simulink library "FloatLibraryOldBlocksBackup"  (R2019a)
settings: Solver=VariableStepAuto  StartTime=0.0  StopTime=10.0  RelTol=1e-3
libraries: arduinolib x2, dspstat3 x2, $bdroot x1
settings Model: Creator=Peter  LastModifiedBy=Peter

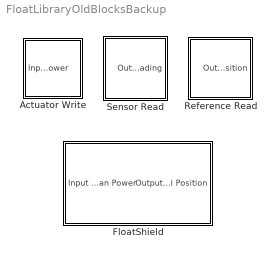
== system FloatLibraryOldBlocksBackup ==
  Actuator Write : Subsystem
      mask DialogControl DescGroupVar Prompt: FloatShield Fan
      mask DialogControl DescTextVar Prompt: Sets power level to the rotating fan at the bottom of the FloatShield tube. Expects input in form of percentual value from 0% to 100%.
      mask Display: image('assets\Fan.svg');
  FloatShield : Subsystem  mask{OutRadio=Percentage (%), Tcal=10, Ts=0.025}
      mask prompts: OutRadio "Output type"; Tcal "Calibration time (s):"; Ts "Sampling period (s):"
      mask init:
      | if OutRadio==1
      |     SatMin=0;
      |     SatMax=100;
      | else
      |     SatMin=0;
      |     SatMax=350;
      | end
      mask TypeOptions OutRadio: Percentage (%) | Altitude (mm)
      mask DialogControl DescGroupVar Prompt: FloatShield
      mask DialogControl DescTextVar Prompt: The block represents the FloatShield device. It accepts an input signal in the range of 0-100% that controls the fan power level and outputs ball position in form selected by the user. The block requires a sampling period and a calibration time at the beginning of the experiment to find out the reading extreme values.
      mask Display: image('assets\FloatShield.svg');
  Reference Read : Subsystem  mask{ReadoutRadio=Percentage (%), Ts=0.025}
      mask prompts: ReadoutRadio "Readout type"; Ts "Sampling period (s):"
      mask init:
      | if ReadoutRadio==1 
      | GainVal = (100/1023);                               
      | elseif ReadoutRadio==2
      | GainVal = (5/1023);                     
      | else
      | GainVal = 1;             
      | end
      mask TypeOptions ReadoutRadio: Percentage (%) | Voltage (V) | Analog value (ADC)
      mask DialogControl DescGroupVar Prompt: FloatShield Potentiometer
      mask DialogControl DescTextVar Prompt: The block represents potentiometer runner on the FloatShield device. User can choose the form of block output that represents the current potentiometer runner position.
      mask Display: image('assets\Potentiometer.svg');
  Sensor Read : Subsystem  mask{OutRadio=Distance (mm), CalType=Default values (recommended), MinVal=15, MaxVal=345, Ts=0.025}
      mask prompts: OutRadio "Output type"; CalType "Calibration values:"; MinVal "Minimal reading (mm):"; MaxVal "Maximal reading (mm):"; Ts "Sampling period (s):"
      mask init:
      | if CalType==1
      |     MinVal=15;
      |     MaxVal=345;
      | end
      | 
      | if OutRadio==2
      |     Rng=MaxVal-MinVal;    
      |     SatMin=0;
      |     SatMax=MaxVal;    
      | else   
      |     Rng=100;
      |     SatMin=0;
      |     SatMax=100;
      | end
      mask TypeOptions OutRadio: Distance (mm) | Altitude (mm) | Percentage (%)
      mask Callback OutRadio:
      | CurrentBlock = gcb;
      | Output = get_param(CurrentBlock,'OutRadio')
      | Calib = get_param(CurrentBlock,'CalType')
      | Menu = Simulink.Mask.get(CurrentBlock);
      | CalibOpt = Menu.getParameter('CalType')
      | MinOpt = Menu.getParameter('MinVal');
      | MaxOpt = Menu.getParameter('MaxVal')
      | 
      | if strcmp(Output,'Distance (mm)')
      | CalibOpt.Enabled='off';
      | MinOpt.Enabled='off';
      | MaxOpt.Enabled='off';
      | elseif strcmp(Calib,'Manual values')
      | CalibOpt.Enabled='on';
      | MinOpt.Enabled='on';
      | MaxOpt.Enabled='on';
      | else
      | CalibOpt.Enabled='on';
      | MinOpt.Enabled='off';
      | MaxOpt.Enabled='off';
      | end
      mask TypeOptions CalType: Default values (recommended) | Manual values
      mask Callback CalType:
      | CurrentBlock = gcbh;
      | Output = get_param(CurrentBlock,'OutRadio');
      | Calib = get_param(CurrentBlock,'CalType');
      | Menu = Simulink.Mask.get(CurrentBlock);
      | MinOpt = Menu.getParameter('MinVal');
      | MaxOpt = Menu.getParameter('MaxVal');
      | 
      | if strcmp(Output,'Distance (mm)')
      | MinOpt.Enabled='off';
      | MaxOpt.Enabled='off';
      | elseif strcmp(Calib,'Manual values')
      | MinOpt.Enabled='on';
      | MaxOpt.Enabled='on';
      | else
      | MinOpt.Enabled='off';
      | MaxOpt.Enabled='off';
      | end
      mask DialogControl DescGroupVar Prompt: FloatShield Distance Sensor
      mask DialogControl DescTextVar Prompt: The block represents the I2C Time of Flight VL53L0X Distance Sensor on the FloatShield device. User can choose type of reading this block outputs. For Altitude or Percentage output, calibration values are required. By default the most probable values are used, but if needed they can be manually set. User can also specify sampling period in seconds.
      mask DialogControl MinVal Tooltip: Recommended 15 mm.
      mask DialogControl MaxVal Tooltip: Recommended 345 mm.
      mask Display: image('assets\TOF.svg');

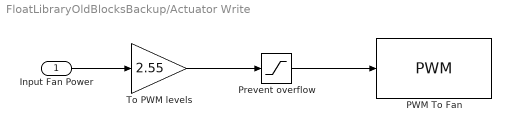
== system FloatLibraryOldBlocksBackup/Actuator Write ==
  Input Fan Power : Inport
  PWM To Fan : arduinolib/PWM  pinNumber=3  EnableInputFrequency=off  InitialFrequency=2000  InitialDutyCycle=0  NotificationType=None  blockPlatform=arduino
  Prevent overflow : Saturate  UpperLimit=255  LowerLimit=0
  To PWM levels : Gain  Gain=2.55
  wires:
  Prevent overflow/1 -> PWM To Fan/1
  To PWM levels/1 -> Prevent overflow/1
  Input Fan Power/1 -> To PWM levels/1

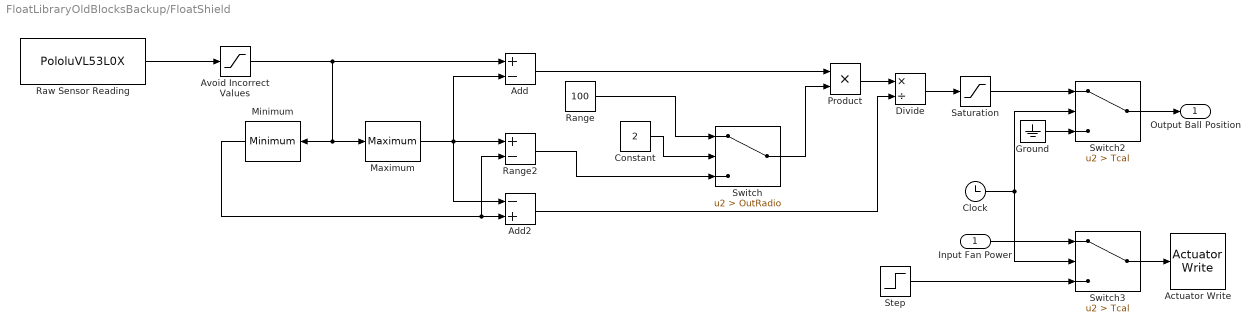
== system FloatLibraryOldBlocksBackup/FloatShield ==
  Input Fan Power : Inport
  Actuator Write : $bdroot/Actuator Write
  Add : Sum  Inputs=+-
  Add2 : Sum  Inputs=-+
  Avoid Incorrect Values : Saturate  UpperLimit=345  LowerLimit=15
  Clock : Clock
  Constant : Constant  Value=2  SampleTime=Ts
  Divide : Product  Inputs=*/
  Ground : Ground
  Maximum : dspstat3/Maximum  operation=maximum  fcn=Running  indexBase=One  operateOver=Each column  Dimension=1  reset=None  roiEnable=off  roiType=Rectangles  roiPortion=Entire ROI  roiOutput=Individual statistics for each ROI  roiFlag=off  roundingMode=Floor  overflowMode=off  accumDataTypeStr=Inherit: Same as product output  accumLastDataTypeStr=Inherit: Same as product output
  Minimum : dspstat3/Minimum  operation=minimum  fcn=Running  indexBase=One  operateOver=Each column  Dimension=1  reset=None  roiEnable=off  roiType=Rectangles  roiPortion=Entire ROI  roiOutput=Individual statistics for each ROI  roiFlag=off  roundingMode=Floor  overflowMode=off
      settings: SourceProductName=DSP System Toolbox  SourceProductBaseCode=DS
  Product : Product
  Range : Constant  Value=100  SampleTime=Ts
  Range2 : Sum  Inputs=+-
  Raw Sensor Reading : S-Function  FunctionName=PololuVL53L0X  SFunctionModules='PololuVL53L0X_wrapper'  SFunctionDeploymentMode=off  EnableBusSupport=off
  Saturation : Saturate  UpperLimit=SatMax  LowerLimit=SatMin
  Step : Step  Time=round((Tcal/2)/Ts)*Ts  After=100  SampleTime=Ts
  Switch : Switch  Criteria=u2 > Threshold  Threshold=OutRadio
  Switch2 : Switch  Criteria=u2 > Threshold  Threshold=Tcal
  Switch3 : Switch  Criteria=u2 > Threshold  Threshold=Tcal
  Output Ball Position : Outport
  wires:
  Range/1 -> Switch/1
  Range2/1 -> Switch/3
  Constant/1 -> Switch/2
  Switch2/1 -> Output Ball Position/1
  Input Fan Power/1 -> Switch3/1
  Switch3/1 -> Actuator Write/1
  Ground/1 -> Switch2/3
  Product/1 -> Divide/1
  Saturation/1 -> Switch2/1
  Avoid Incorrect Values/1 -> Add/1, Maximum/1, Minimum/1
  Add2/1 -> Divide/2
  Divide/1 -> Saturation/1
  Raw Sensor Reading/1 -> Avoid Incorrect Values/1
  Step/1 -> Switch3/3
  Minimum/1 -> Add2/2, Range2/2
  Clock/1 -> Switch3/2, Switch2/2
  Maximum/1 -> Add2/1, Add/2, Range2/1
  Add/1 -> Product/1
  Switch/1 -> Product/2

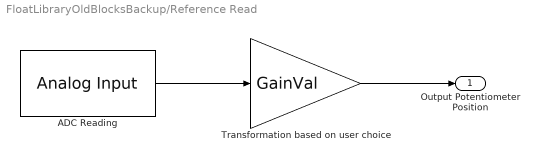
== system FloatLibraryOldBlocksBackup/Reference Read ==
  ADC Reading : arduinolib/Analog Input  pinNumber=0  ReadResultsOnly=off  ConversionTriggerSource=Software  ExternalTriggerType=uint32(0)  OutputDataType=uint16  EnableConversionCompleteNotify=off  EnableOuputStatus=off  SampleTime=Ts  blockPlatform=arduino
  Transformation based on user choice : Gain  Gain=GainVal  ParamDataTypeStr=double
  "Output Potentiometer Position " : Outport
  wires:
  ADC Reading/1 -> Transformation based on user choice/1
  Transformation based on user choice/1 -> "Output Potentiometer Position "/1

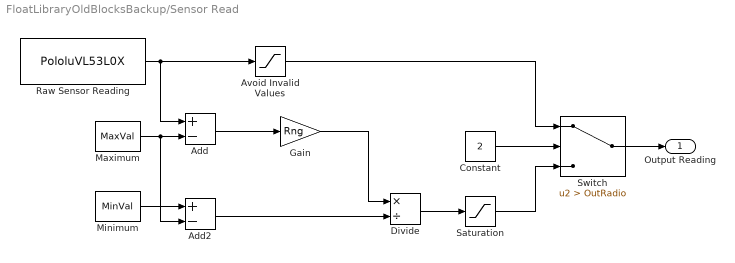
== system FloatLibraryOldBlocksBackup/Sensor Read ==
  Add : Sum  Inputs=+-
  Add2 : Sum  Inputs=+-
  Avoid Invalid Values : Saturate  UpperLimit=350  LowerLimit=10
  Constant : Constant  Value=2  SampleTime=Ts
  Divide : Product  Inputs=*/
  Gain : Gain  Gain=Rng
  Maximum : Constant  Value=MaxVal  SampleTime=Ts
  Minimum : Constant  Value=MinVal  SampleTime=Ts
  Raw Sensor Reading : S-Function  FunctionName=PololuVL53L0X  SFunctionModules='PololuVL53L0X_wrapper'  SFunctionDeploymentMode=off  EnableBusSupport=off
  Saturation : Saturate  UpperLimit=SatMax  LowerLimit=SatMin
  Switch : Switch  Criteria=u2 > Threshold  Threshold=OutRadio
  Output Reading : Outport  SampleTime=Ts
  wires:
  Saturation/1 -> Switch/3
  Gain/1 -> Divide/1
  Avoid Invalid Values/1 -> Switch/1
  Switch/1 -> Output Reading/1
  Divide/1 -> Saturation/1
  Add/1 -> Gain/1
  Add2/1 -> Divide/2
  Minimum/1 -> Add2/1
  Constant/1 -> Switch/2
  Maximum/1 -> Add2/2, Add/2
  Raw Sensor Reading/1 -> Avoid Invalid Values/1, Add/1
